simulink model "fofb"  (Simulink 7.8)
settings: Solver=ode45  StartTime=0.0  StopTime=1e-1  RelTol=1e-3
values from neighbouring files (symbols this model uses):
  simparam = struct(     'beam', beam,      'distbeam', distbeam,      'fofbctrl', fofbctrl,      'bpm', bpm,      'dcct', dcct,      'psctrl', psctrl,      'psfilter', psfilter,      'corrmagnet', corrmagnet,      'vacchamb', vacchamb,      'simvectors', simvectors)    [simfofb.m]
settings Model: Creator=daniel.tavares  LastModifiedBy=daniel.tavares
settings DataIOCC: ExternalInput=[simparam.simvectors.t simparam.simvectors.dist simparam.simvectors.bpm_noise simparam.simvectors.dcct_noise simparam.simvectors.psoutput_noise]  LimitDataPoints=off  LoadExternalInput=on  SaveState=on  SignalLogging=off  DSMLogging=off

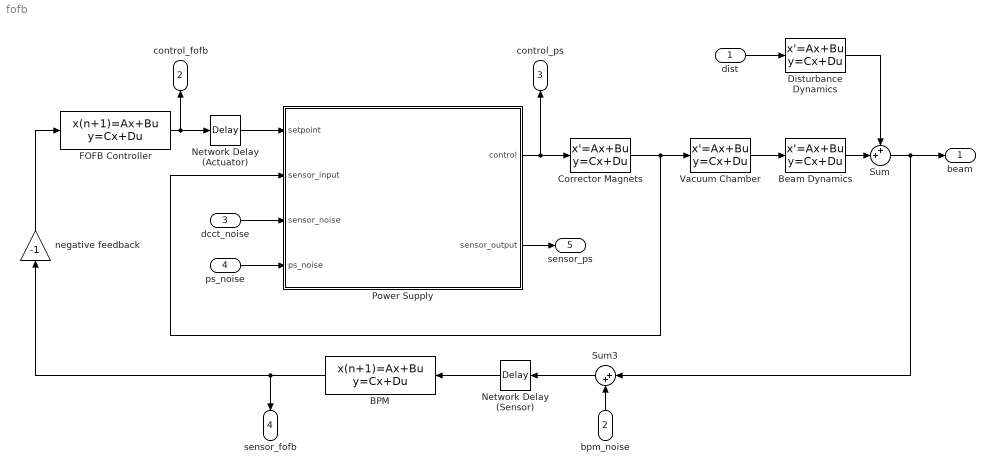
== system fofb ==
  dist : Inport  PortDimensions=size(simparam.distbeam.d, 2)
  bpm_noise : Inport  Port=2  PortDimensions=size(simparam.beam.d, 1)
  dcct_noise : Inport  Port=3  PortDimensions=size(simparam.beam.d, 2)
  ps_noise : Inport  Port=4  PortDimensions=size(simparam.beam.d, 2)
  BPM : DiscreteStateSpace  A=simparam.bpm.a  B=simparam.bpm.b  C=simparam.bpm.c  D=simparam.bpm.d  SampleTime=simparam.bpm.Ts
  Beam Dynamics : StateSpace  A=simparam.beam.a  B=simparam.beam.b  C=simparam.beam.c  D=simparam.beam.d
  Corrector Magnets : StateSpace  A=simparam.corrmagnet.a  B=simparam.corrmagnet.b  C=simparam.corrmagnet.c  D=simparam.corrmagnet.d
  Disturbance Dynamics : StateSpace  A=simparam.distbeam.a  B=simparam.distbeam.b  C=simparam.distbeam.c  D=simparam.distbeam.d
  FOFB Controller : DiscreteStateSpace  A=simparam.fofbctrl.a  B=simparam.fofbctrl.b  C=simparam.fofbctrl.c  D=simparam.fofbctrl.d  SampleTime=simparam.fofbctrl.Ts
  Network Delay (Actuator) : TransportDelay  DelayTime=repmat(simparam.fofbctrl.actdelay, 1, size(simparam.beam.d, 2))
  Network Delay (Sensor) : TransportDelay  DelayTime=repmat(simparam.fofbctrl.sensdelay, 1, size(simparam.beam.d, 1))
  Power Supply : Subsystem
  Sum : Sum  Inputs=++|
  Sum3 : Sum  Inputs=|++
  Vacuum Chamber : StateSpace  A=simparam.vacchamb.a  B=simparam.vacchamb.b  C=simparam.vacchamb.c  D=simparam.vacchamb.d
  negative feedback : Gain  Gain=-1
  beam : Outport
  control_fofb : Outport  Port=2
  control_ps : Outport  Port=3
  sensor_fofb : Outport  Port=4
  sensor_ps : Outport  Port=5
  wires:
  Corrector Magnets/1 -> Vacuum Chamber/1, Power Supply/2(sensor_input)
  FOFB Controller/1 -> control_fofb/1, Network Delay (Actuator)/1
  Beam Dynamics/1 -> Sum/2
  dist/1 -> Disturbance Dynamics/1
  bpm_noise/1 -> Sum3/2
  ps_noise/1 -> Power Supply/4(ps_noise)
  dcct_noise/1 -> Power Supply/3(sensor_noise)
  Power Supply/1(control) -> control_ps/1, Corrector Magnets/1
  Power Supply/2(sensor_output) -> sensor_ps/1
  Sum3/1 -> Network Delay (Sensor)/1
  BPM/1 -> sensor_fofb/1, negative feedback/1
  negative feedback/1 -> FOFB Controller/1
  Network Delay (Actuator)/1 -> Power Supply/1(setpoint)
  Network Delay (Sensor)/1 -> BPM/1
  Vacuum Chamber/1 -> Beam Dynamics/1
  Disturbance Dynamics/1 -> Sum/1
  Sum/1 -> beam/1, Sum3/1

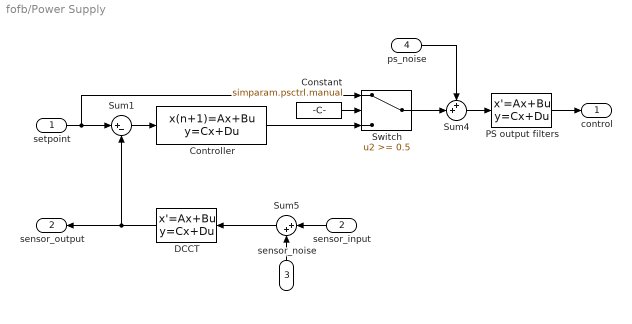
== system fofb/Power Supply ==
  setpoint : Inport
  sensor_input : Inport  Port=2
  sensor_noise : Inport  Port=3
  ps_noise : Inport  Port=4
  Constant : Constant  Value=simparam.psctrl.manual
  Controller : DiscreteStateSpace  A=simparam.psctrl.a  B=simparam.psctrl.b  C=simparam.psctrl.c  D=simparam.psctrl.d  SampleTime=simparam.psctrl.Ts
  DCCT : StateSpace  A=simparam.dcct.a  B=simparam.dcct.b  C=simparam.dcct.c  D=simparam.dcct.d
  PS output filters : StateSpace  A=simparam.psfilter.a  B=simparam.psfilter.b  C=simparam.psfilter.c  D=simparam.psfilter.d
  Sum1 : Sum  Inputs=|+-
  Sum4 : Sum  Inputs=++|
  Sum5 : Sum  Inputs=|++
  Switch : Switch  Threshold=0.5
  control : Outport
  sensor_output : Outport  Port=2
  wires:
  Sum1/1 -> Controller/1
  setpoint/1 -> Sum1/1, Switch/1
  Switch/1 -> Sum4/2
  Sum4/1 -> PS output filters/1
  ps_noise/1 -> Sum4/1
  sensor_noise/1 -> Sum5/2
  Sum5/1 -> DCCT/1
  DCCT/1 -> sensor_output/1, Sum1/2
  sensor_input/1 -> Sum5/1
  PS output filters/1 -> control/1
  Controller/1 -> Switch/3
  Constant/1 -> Switch/2
